simulink model "s_pol5"  (Simulink 8.1)
settings: Solver=ode45  SolverMode=SingleTasking  StartTime=0.0  StopTime=10  MaxStep=0.10  RelTol=1e-3  AbsTol=1e-6
values from neighbouring files (symbols this model uses):
  K = lqrd(A, B, Q, R, Ts)    [abeob1.m]    (also in apol1.m = place(A, B, p); kalm3.m = K*0; kalm4.m = K_temp; lqr_2.m = place(A',C',p))
  ki = 0.8/ks    [pol4.m]    (also in pol5.m = -Kn(n+1); pol7.m = -Kn(n+1))
undefined symbols (not defined in the file): A, B, C
settings Model: Creator=mainster  LastModifiedBy=mainster
settings DataIOCC: LimitDataPoints=off  SaveOutput=off  SaveTime=off
settings OptimizationCC: BlockReduction=off  BooleanDataType=off  ExpressionDepthLimit=128
settings DebuggingCC: SaveWithParameterizedLinksMsg=none  SignalResolutionControl=TryResolveAllWithWarning  SolverPrmCheckMsg=none  MultiTaskDSMMsg=warning  MultiTaskCondExecSysMsg=none  FcnCallInpInsideContextMsg=EnableAllAsError  StrictBusMsg=None
settings HardwareCC: TargetUnknown=on
settings RTWCC: IncludeERTFirstTime=on

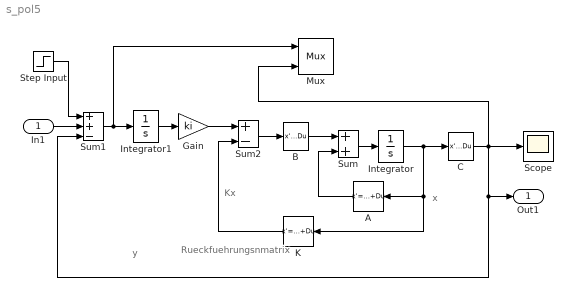
== system s_pol5 ==
  note: Kx
  note: Rueckfuehrungsnmatrix
  note: x
  note: y
  In1 : Inport
  A : StateSpace  A=[]  B=[]  C=[]  D=K  mask(Matrix Gain){K=A}
      mask prompts: K "Gain matrix:"
      mask help: Matrix Gain.
      mask Help: Multiplies input vector by entered matrix to produce output vector (y=Au).
      mask Display: disp('K')
  B : StateSpace  A=[]  B=[]  C=[]  D=K  mask(Matrix Gain){K=B}
      mask prompts: K "Gain matrix:"
      mask help: Matrix Gain.
      mask Help: Multiplies input vector by entered matrix to produce output vector (y=Au).
      mask Display: disp('K')
  C : StateSpace  A=[]  B=[]  C=[]  D=K  mask(Matrix Gain){K=C}
      mask prompts: K "Gain matrix:"
      mask help: Matrix Gain.
      mask Help: Multiplies input vector by entered matrix to produce output vector (y=Au).
      mask Display: disp('K')
  Gain : Gain  Gain=ki  SaturateOnIntegerOverflow=on  OutDataTypeStr=Inherit: Same as input  ParamDataTypeStr=Inherit: Same as input
  Integrator : Integrator
  Integrator1 : Integrator
  K : StateSpace  A=[]  B=[]  C=[]  D=K  mask(Matrix Gain){K=K}
      mask prompts: K "Gain matrix:"
      mask help: Matrix Gain.
      mask Help: Multiplies input vector by entered matrix to produce output vector (y=Au).
      mask Display: disp('K')
  Mux : Mux  Inputs=2
  Scope : Scope
      settings: TickLabels=on  TimeRange=12.060000  YMin=-20000.000000  YMax=20000.000000
  Step Input : Step  Time=0  SampleTime=0
  Sum : Sum  SaturateOnIntegerOverflow=on  InputSameDT=on  OutDataTypeStr=Inherit: Same as first input
  Sum1 : Sum  Inputs=++-  SaturateOnIntegerOverflow=on  InputSameDT=on  OutDataTypeStr=Inherit: Same as first input
  Sum2 : Sum  Inputs=+-  SaturateOnIntegerOverflow=on  InputSameDT=on  OutDataTypeStr=Inherit: Same as first input
  Out1 : Outport
  wires:
  Sum1/1 -> Mux/1, Integrator1/1
  Gain/1 -> Sum2/1
  Integrator1/1 -> Gain/1
  C/1 -> Mux/2, Scope/1, Sum1/3, Out1/1
  Integrator/1 -> A/1, K/1, C/1
  K/1 -> Sum2/2
  Sum2/1 -> B/1
  A/1 -> Sum/2
  Sum/1 -> Integrator/1
  B/1 -> Sum/1
  In1/1 -> Sum1/2
  Step Input/1 -> Sum1/1
